simulink model "hw6_pr3"  (Simulink 7.3)
settings: Solver=ode45  StartTime=0.0  StopTime=100  MaxStep=0.1  RelTol=1e-3
values from neighbouring files (symbols this model uses):
  A1 = [-4 5; -1 -2]    [GlobalL2L2GainEx1.m]
  A2 = [3 6 3; 1 2 1]/4    [GlobalL2L2GainEx1.m]
  A3 = [-1 0 -9 6; 0 -3 6 -7]/8    [GlobalL2L2GainEx1.m]
  B = [10 2; 0 1]    [GlobalL2L2GainEx1.m]
  C = [1 1; 2 3]    [GlobalL2L2GainEx1.m]
  X0 = [0;0]    [GlobalL2L2GainEx1.m]
settings Model: Creator=pjseiler  LastModifiedBy=pjseiler

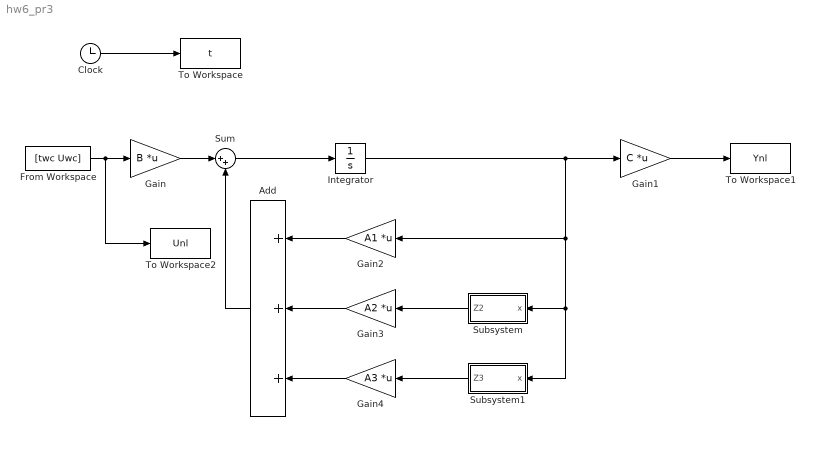
== system hw6_pr3 ==
  Add : Sum  Inputs=+++  OutDataType=fixdt(1, 16)  OutScaling=2^-10
  Clock : Clock
      settings: Decimation=10
  From Workspace : FromWorkspace  VariableName=[twc Uwc]  SampleTime=0
  Gain : Gain  Gain=B  Multiplication=Matrix(K*u)  ParameterDataType=fixdt(1, 16)  ParameterScaling=2^0  OutDataType=fixdt(1, 16)  OutScaling=2^0
  Gain1 : Gain  Gain=C  Multiplication=Matrix(K*u)  ParameterDataType=fixdt(1, 16)  ParameterScaling=2^0  OutDataType=fixdt(1, 16)  OutScaling=2^0
  Gain2 : Gain  Gain=A1  Multiplication=Matrix(K*u)  ParameterDataType=fixdt(1, 16)  ParameterScaling=2^0  OutDataType=fixdt(1, 16)  OutScaling=2^0
  Gain3 : Gain  Gain=A2  Multiplication=Matrix(K*u)  ParameterDataType=fixdt(1, 16)  ParameterScaling=2^0  OutDataType=fixdt(1, 16)  OutScaling=2^0
  Gain4 : Gain  Gain=A3  Multiplication=Matrix(K*u)  ParameterDataType=fixdt(1, 16)  ParameterScaling=2^0  OutDataType=fixdt(1, 16)  OutScaling=2^0
  Integrator : Integrator  InitialCondition=X0
  Subsystem : Subsystem
  Subsystem1 : Subsystem
  Sum : Sum  Inputs=|++  OutDataType=fixdt(1, 16)  OutScaling=2^0
  To Workspace : ToWorkspace  VariableName=t  SampleTime=-1  SaveFormat=Array
  To Workspace1 : ToWorkspace  VariableName=Ynl  SampleTime=-1  SaveFormat=Array
  To Workspace2 : ToWorkspace  VariableName=Unl  SampleTime=-1  SaveFormat=Array
  wires:
  Clock/1 -> To Workspace/1
  From Workspace/1 -> Gain/1, To Workspace2/1
  Gain/1 -> Sum/1
  Sum/1 -> Integrator/1
  Integrator/1 -> Gain1/1, Gain2/1, Subsystem/1(x), Subsystem1/1(x)
  Gain1/1 -> To Workspace1/1
  Gain2/1 -> Add/1
  Add/1 -> Sum/2
  Gain3/1 -> Add/2
  Gain4/1 -> Add/3
  Subsystem/1(Z2) -> Gain3/1
  Subsystem1/1(Z3) -> Gain4/1

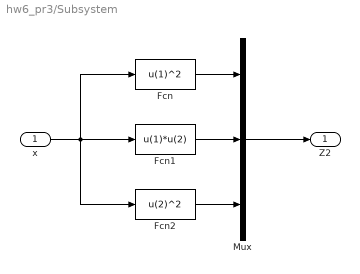
== system hw6_pr3/Subsystem ==
  x : Inport  OutDataType=fixdt(1, 16)  OutScaling=2^0
  Fcn : Fcn  Expr=u(1)^2
  Fcn1 : Fcn  Expr=u(1)*u(2)
  Fcn2 : Fcn  Expr=u(2)^2
  Mux : Mux  Inputs=3
  Z2 : Outport  OutDataType=fixdt(1, 16)  OutScaling=2^0
  wires:
  x/1 -> Fcn1/1, Fcn2/1, Fcn/1
  Fcn/1 -> Mux/1
  Fcn1/1 -> Mux/2
  Fcn2/1 -> Mux/3
  Mux/1 -> Z2/1

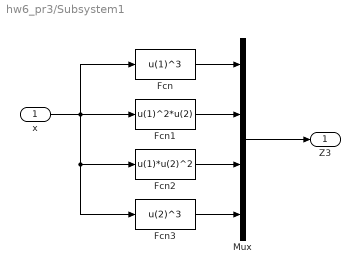
== system hw6_pr3/Subsystem1 ==
  x : Inport  OutDataType=fixdt(1, 16)  OutScaling=2^0
  Fcn : Fcn  Expr=u(1)^3
  Fcn1 : Fcn  Expr=u(1)^2*u(2)
  Fcn2 : Fcn  Expr=u(1)*u(2)^2
  Fcn3 : Fcn  Expr=u(2)^3
  Mux : Mux
  Z3 : Outport  OutDataType=fixdt(1, 16)  OutScaling=2^0
  wires:
  Mux/1 -> Z3/1
  Fcn2/1 -> Mux/3
  Fcn1/1 -> Mux/2
  Fcn/1 -> Mux/1
  x/1 -> Fcn/1, Fcn1/1, Fcn2/1, Fcn3/1
  Fcn3/1 -> Mux/4
